simulink model "VTOL_sim"  (R2015a)
settings: Solver=ode45  StartTime=0.0  StopTime=10000  RelTol=1e-3
InitFcn:
  | param
undefined symbols (not defined in the file or in its folder): drawVTOL
libraries: simulink x3
settings Model: Creator=beard  LastModifiedBy=jhl48
settings DataIOCC: SignalLoggingSaveFormat=ModelDataLogs
settings OptimizationCC: ExpressionDepthLimit=2147483647  InitFltsAndDblsToZero=on
settings DebuggingCC: UnderspecifiedInitializationDetection=Classic  MergeDetectMultiDrivingBlocksExec=none  SolverPrmCheckMsg=warning  FcnCallInpInsideContextMsg=UseLocalSettings  StateNameClashWarn=warning
settings GRTTargetCC: CombineOutputUpdateFcns=off  GRTInterface=on

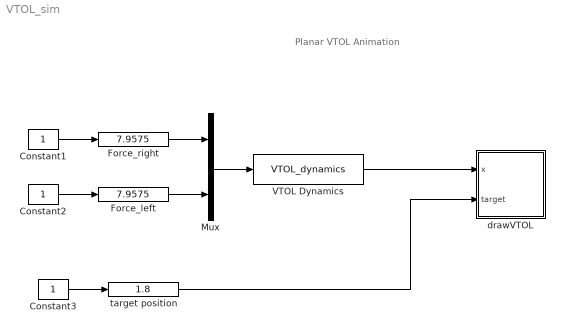
== system VTOL_sim ==
  note: Planar VTOL Animation
  Constant1 : Constant
  Constant2 : Constant
  Constant3 : Constant
  Force_left : simulink/Math Operations/Slider Gain  low=-10  gain=7.9575  high=50
  Force_right : simulink/Math Operations/Slider Gain  low=-10  gain=7.9575  high=50
  Mux : Mux  Inputs=2
  VTOL Dynamics : S-Function  FunctionName=VTOL_dynamics  Parameters=AP
  drawVTOL : Subsystem
      mask Display: image(imread('tv.jpg'))
  target position : simulink/Math Operations/Slider Gain  low=-10  gain=1.8  high=50
  wires:
  Constant1/1 -> Force_right/1
  Mux/1 -> VTOL Dynamics/1
  Force_right/1 -> Mux/1
  Constant2/1 -> Force_left/1
  Force_left/1 -> Mux/2
  Constant3/1 -> target position/1
  VTOL Dynamics/1 -> drawVTOL/1(x)
  target position/1 -> drawVTOL/2(target)

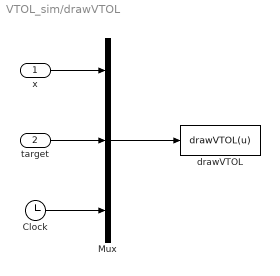
== system VTOL_sim/drawVTOL ==
  x : Inport
  target : Inport  Port=2
  Clock : Clock
  Mux : Mux  Inputs=3
  drawVTOL : MATLABFcn  MATLABFcn=drawVTOL(u)  OutputDimensions=0  SampleTime=0.001
  wires:
  Mux/1 -> drawVTOL/1
  x/1 -> Mux/1
  Clock/1 -> Mux/3
  target/1 -> Mux/2
